simulink model "Controller"  (R2020b)
settings: Solver=VariableStepAuto  StartTime=0.0  StopTime=50  RelTol=1e-3
settings Model: Creator=Awan  LastModifiedBy=Awan
settings SolverCC: ZeroCrossAlgorithm=Adaptive
settings DebuggingCC: IgnoredZcDiagnostic=none

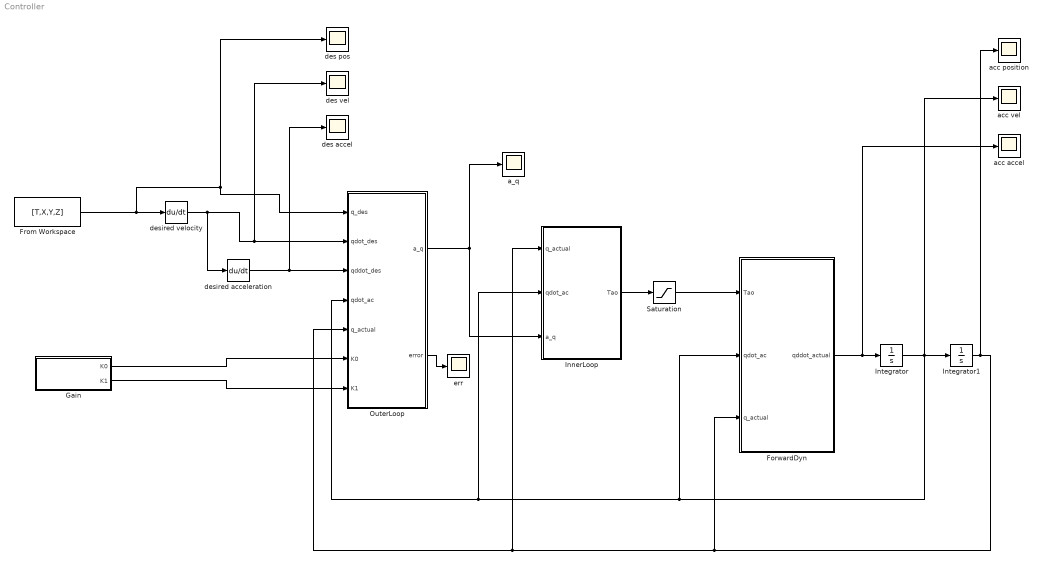
== system Controller ==
  ForwardDyn : MATLAB Function  TreatAsAtomicUnit=on
  From Workspace : FromWorkspace  VariableName=[T,X,Y,Z]
  Gain : Subsystem
  InnerLoop : MATLAB Function  TreatAsAtomicUnit=on
  Integrator : Integrator  InitialCondition=[0,0,0]
  Integrator1 : Integrator  InitialCondition=[0,0,0]
  OuterLoop : MATLAB Function  TreatAsAtomicUnit=on
  Saturation : Saturate  UpperLimit=6000  LowerLimit=-6000  ZeroCross=off
  a_q : Scope
  acc accel : Scope
  acc position : Scope
  acc vel : Scope
  des accel : Scope
  des pos : Scope
  des vel : Scope
  desired acceleration : Derivative
  desired velocity : Derivative
  err : Scope
  wires:
  desired acceleration/1 -> des accel/1, OuterLoop/3(qddot_des)
  desired velocity/1 -> desired acceleration/1, des vel/1, OuterLoop/2(qdot_des)
  Gain/1(K0) -> OuterLoop/6(K0)
  Gain/2(K1) -> OuterLoop/7(K1)
  OuterLoop/2(error) -> err/1
  From Workspace/1 -> des pos/1, OuterLoop/1(q_des), desired velocity/1
  OuterLoop/1(a_q) -> a_q/1, InnerLoop/3(a_q)
  InnerLoop/1(Tao) -> Saturation/1
  Saturation/1 -> ForwardDyn/1(Tao)
  ForwardDyn/1(qddot_actual) -> acc accel/1, Integrator/1
  Integrator/1 -> Integrator1/1, acc vel/1, InnerLoop/2(qdot_ac), OuterLoop/4(qdot_ac), ForwardDyn/2(qdot_ac)
  Integrator1/1 -> InnerLoop/1(q_actual), OuterLoop/5(q_actual), ForwardDyn/3(q_actual), acc position/1

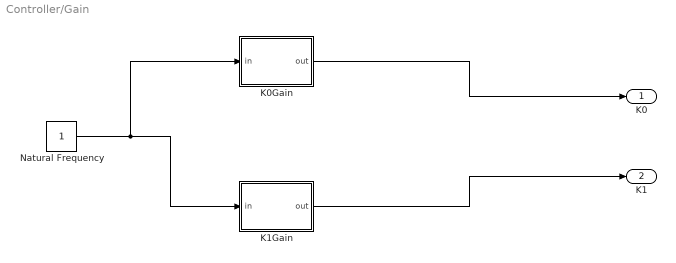
== system Controller/Gain ==
  K0Gain : MATLAB Function  TreatAsAtomicUnit=on
  K1Gain : MATLAB Function  TreatAsAtomicUnit=on
  Natural Frequency : Constant
  K0 : Outport
  K1 : Outport  Port=2  VectorParamsAs1DForOutWhenUnconnected=off
  wires:
  K1Gain/1(out) -> K1/1
  K0Gain/1(out) -> K0/1
  Natural Frequency/1 -> K1Gain/1(in), K0Gain/1(in)

== matlab function Controller/Gain/K1Gain ==
  data: in input; out output
function out = K1Gain(in)
%gain adjustment for K1
in=0.7*in;

out=[in, 0, 0; 0, in, 0; 0, 0, in];

== matlab function Controller/OuterLoop ==
  data: q_des input; a_q output; qdot_des input; qddot_des input; qdot_ac input; q_actual input; K0 input; K1 input; error output
function [a_q,error] = control(q_des,qdot_des,qddot_des,qdot_ac,q_actual,K0,K1)
%Linear System Stabilizer/Outer Loop Controller 

q_squig=(q_actual - q_des);
qdot_squig=(qdot_ac-qdot_des);

a_q = (qddot_des)-(K0*q_squig)-(K1*qdot_squig);
error = [q_des-q_actual];

== matlab function Controller/Gain/K0Gain ==
  data: in input; out output
function out = K0Gain(in)
%gain adjustment for K0
in=0.3*in;

out=[in, 0, 0; 0, in, 0; 0, 0, in];

== matlab function Controller/InnerLoop ==
  data: q_actual input; qdot_ac input; a_q input; Tao output
function Tao=dyneqoutloop(q_actual,qdot_ac,a_q) 
%Function that calculates Torques based on the Euler Lagrange Method
%Now Modified for Inner Loop
%************************************************************************
%Code Section 1: Input Parameters 
%************************************************************************
m= [945.89, 480.13, 112.70]; %mass per link (g) 
L= [1.5, 1.75, 0.3]; %link lengths (m) 
L_c=[0.65, 0.84, 0.17]; %distances from link start to centre of mass (m)
g=9.81; %grav constant 
%intertia matrices about centre of masses
I1=[ 196.52, 0, 0; 0, 53.6, 0; 0, 0, 191.83 ];
I2=[ 8.41, 0, 0; 0, 144.37, 0; 0, 0, 147.97 ];
I3=[ 3.52, 0, 0; 0, 5.10, 0; 0, 0, 3.15 ];
%************************************************************************
%Code Section 2: Computing DH Matrices 
%************************************************************************
%DH Parameters 
a = [0, L(2), L(3)]; %a values 
d = [L(1), 0, 0]; %d values 
a_c = [0, L_c(2), L_c(3)]; %a values, modified for centre of mass
d_c = [L_c(1), 0, 0]; %d values, modified for centre of mass
alpha = [-pi/2, 0, 0]; %alpha angles
theta = [q_actual(1), q_actual(2), q_actual(3)]; %joint angles
%Regulr DH Matrices  
A1= [ cos(theta(1)), -sin(theta(1)) * cosd(alpha(1)*(180/pi)), sin(theta(1))*sind(alpha(1)*(180/pi)), a(1)*cos(theta(1)); 
            sin(theta(1)), cos(theta(1))*cosd(alpha(1)*(180/pi)), -cos(theta(1))*sind(alpha(1)*(180/pi)), a(1)*sin(theta(1));
            0, sind(alpha(1)*(180/pi)), cosd(alpha(1)*(180/pi)), d(1); 
            0, 0, 0, 1; ]; 
        
Temp_A2= [ cos(theta(2)), -sin(theta(2)) * cosd(alpha(2)*(180/pi)), sin(theta(2))*sind(alpha(2)*(180/pi)), a(2)*cos(theta(2)); 
            sin(theta(2)), cos(theta(2))*cosd(alpha(2)*(180/pi)), -cos(theta(2))*sind(alpha(2)*(180/pi)), a(2)*sin(theta(2));
            0, sind(alpha(2)*(180/pi)), cosd(alpha(2)*(180/pi)), d(2); 
            0, 0, 0, 1; ]; 
        
%Modded DH Matrices  
Ac1= [ cos(theta(1)), -sin(theta(1)) * cosd(alpha(1)*(180/pi)), sin(theta(1))*sind(alpha(1)*(180/pi)), a_c(1)*cos(theta(1)); 
            sin(theta(1)), cos(theta(1))*cosd(alpha(1)*(180/pi)), -cos(theta(1))*sind(alpha(1)*(180/pi)), a_c(1)*sin(theta(1));
            0, sind(alpha(1)*(180/pi)), cosd(alpha(1)*(180/pi)), d_c(1); 
            0, 0, 0, 1; ] ;
             
Temp_Ac2= [ cos(theta(2)), -sin(theta(2)) * cosd(alpha(2)*(180/pi)), sin(theta(2))*sind(alpha(2)*(180/pi)), a_c(2)*cos(theta(2)); 
            sin(theta(2)), cos(theta(2))*cosd(alpha(2)*(180/pi)), -cos(theta(2))*sind(alpha(2)*(180/pi)), a_c(2)*sin(theta(2));
            0, sind(alpha(2)*(180/pi)), cosd(alpha(2)*(180/pi)), d_c(2); 
            0, 0, 0, 1; ] ;        
        
Temp_Ac3= [ cos(theta(3)), -sin(theta(3)) * cosd(alpha(3)*(180/pi)), sin(theta(3))*sind(alpha(3)*(180/pi)), a_c(3)*cos(theta(3)); 
            sin(theta(3)), cos(theta(3))*cosd(alpha(3)*(180/pi)), -cos(theta(3))*sind(alpha(3)*(180/pi)), a_c(3)*sin(theta(3));
            0, sind(alpha(3)*(180/pi)), cosd(alpha(3)*(180/pi)), d_c(3); 
            0, 0, 0, 1; ] ;
%Computing Transformation Matrices
A2=A1*Temp_A2;
Ac2=A1*Temp_Ac2;
Ac3=A1*Temp_A2*Temp_Ac3;
%************************************************************************
%Code Section 3: Computing Jacobian Matrices 
%************************************************************************        
%z vectors
z0=[0 0 1].';
z1= A1(1:3, 3);
z2= A2(1:3, 3);
%origin vectors
o0=[0 0 0].';
o1= A1(1:3, 4);
o2= A2(1:3, 4);
%centre of mass origin vectors 
oc1=Ac1(1:3, 4);
oc2=Ac2(1:3, 4);
oc3=Ac3(1:3, 4);
%Jacobians
J1=[ cross(z0,oc1 - o0), zeros(3,1), zeros(3,1);
     z0, zeros(3,1), zeros(3,1) ];
J2=[ cross(z0,oc2 - o0), cross(z1,oc2 - o1), zeros(3,1);
    z0, z1, zeros(3,1) ];
J3=[ cross(z0,oc3 - o0), cross(z1,oc3 - o1), cross(z2,oc3 - o2);
    z0, z1, z2 ];        
%************************************************************************
%Code Section 4: Computing Linear and Rotational Kinetic Energy
%************************************************************************
%Velocity Jacobians 
Jv1=J1(1:3,1:3);
Jv2=J2(1:3,1:3);
Jv3=J3(1:3,1:3);
%Linear KE Calculation
KL1=m(1)*(Jv1.')*Jv1;
KL2=m(2)*(Jv2.')*Jv2;
KL3=m(3)*(Jv3.')*Jv3;
%************************************************************************
%Rotational Jacobians 
Jw1=J1(4:6,1:3);
Jw2=J2(4:6,1:3);
Jw3=J3(4:6,1:3);
%R values 
R1=Ac1(1:3,1:3);
R2=Ac2(1:3,1:3);
R3=Ac3(1:3,1:3);
%Rotational KE Calculation
KW1=(Jw1.')*R1*I1*(R1.')*Jw1;
KW2=(Jw2.')*R2*I2*(R2.')*Jw2;
KW3=(Jw3.')*R3*I3*(R3.')*Jw3;
%************************************************************************
%Code Section 5: Computing Inertia Matrix
%************************************************************************
%Summing Kinetic Energies
SumKE1=KL1*KW1;
SumKE2=KL2*KW2;
SumKE3=KL3*KW3;
%Formulating D Matrix 
D=SumKE1+SumKE2+SumKE3;
%************************************************************************
%Code Section 6: Computing Christoffel Symbols (Modified and Taken from EulerLagrangeAttempt2.m 
%************************************************************************
%cij1 values 
c111=0;
c221=0;
c331=0;

c121=- 157.7504*sin(2*q_actual(2) + q_actual(3)) - 2.5199e+04*sin(2*q_actual(2)) - 1.1515e+04*sin(4*q_actual(2)) - 144.6372*sin(2*q_actual(2) + 2*q_actual(3)) - 13.2437*sin(2*q_actual(2) + 3*q_actual(3)) - 136.3318*sin(4*q_actual(2) + 2*q_actual(3)) - 26.4873*sin(4*q_actual(2) + 3*q_actual(3)) - 1.2865*sin(4*q_actual(2) + 4*q_actual(3));
c131=- 78.8752*sin(2*q_actual(2) + q_actual(3)) - 68.1659*sin(2*q_actual(3)) - 144.6372*sin(2*q_actual(2) + 2*q_actual(3)) - 19.8655*sin(2*q_actual(2) + 3*q_actual(3)) - 68.1659*sin(4*q_actual(2) + 2*q_actual(3)) - 19.8655*sin(4*q_actual(2) + 3*q_actual(3)) - 1.2865*sin(4*q_actual(2) + 4*q_actual(3)) - 78.8752*sin(q_actual(3));

c211=c121;
c311=c131;

c231=0;
c321=c231;

%cij2 values 
c112=157.7504*sin(2*q_actual(2) + q_actual(3)) + 2.5199e+04*sin(2*q_actual(2)) + 1.1515e+04*sin(4*q_actual(2)) + 144.6372*sin(2*q_actual(2) + 2*q_actual(3)) + 13.2437*sin(2*q_actual(2) + 3*q_actual(3)) + 136.3318*sin(4*q_actual(2) + 2*q_actual(3)) + 26.4873*sin(4*q_actual(2) + 3*q_actual(3)) + 1.2865*sin(4*q_actual(2) + 4*q_actual(3));
c222=0;
c332=-316.8420*sin(q_actual(3));

c122=157.7504*sin(2*q_actual(2) + q_actual(3)) + 2.5199e+04*sin(2*q_actual(2)) + 1.1515e+04*sin(4*q_actual(2)) + 144.6372*sin(2*q_actual(2) + 2*q_actual(3)) + 13.2437*sin(2*q_actual(2) + 3*q_actual(3)) + 136.3318*sin(4*q_actual(2) + 2*q_actual(3)) + 26.4873*sin(4*q_actual(2) + 3*q_actual(3)) + 1.2865*sin(4*q_actual(2) + 4*q_actual(3));
c132=157.7504*sin(2*q_actual(2) + q_actual(3)) + 2.5199e+04*sin(2*q_actual(2)) + 1.1515e+04*sin(4*q_actual(2)) + 144.6372*sin(2*q_actual(2) + 2*q_actual(3)) + 13.2437*sin(2*q_actual(2) + 3*q_actual(3)) + 136.3318*sin(4*q_actual(2) + 2*q_actual(3)) + 26.4873*sin(4*q_actual(2) + 3*q_actual(3)) + 1.2865*sin(4*q_actual(2) + 4*q_actual(3));

c212=c122;
c312=c132;

c232=-158.4210*sin(q_actual(3));
c322=c232;

%cij3 values 
c113=78.8752*sin(2*q_actual(2) + q_actual(3)) + 68.1659*sin(2*q_actual(3)) + 144.6372*sin(2*q_actual(2) + 2*q_actual(3)) + 19.8655*sin(2*q_actual(2) + 3*q_actual(3)) + 68.1659*sin(4*q_actual(2) + 2*q_actual(3)) + 19.8655*sin(4*q_actual(2) + 3*q_actual(3)) + 1.2865*sin(4*q_actual(2) + 4*q_actual(3)) + 78.8752*sin(q_actual(3));
c223=158.4210*sin(q_actual(3));
c333=-52.8070*sin(q_actual(3));

c123=78.8752*sin(2*q_actual(2) + q_actual(3)) + 68.1659*sin(2*q_actual(3)) + 144.6372*sin(2*q_actual(2) + 2*q_actual(3)) + 19.8655*sin(2*q_actual(2) + 3*q_actual(3)) + 68.1659*sin(4*q_actual(2) + 2*q_actual(3)) + 19.8655*sin(4*q_actual(2) + 3*q_actual(3)) + 1.2865*sin(4*q_actual(2) + 4*q_actual(3)) + 78.8752*sin(q_actual(3));
c133=78.8752*sin(2*q_actual(2) + q_actual(3)) + 68.1659*sin(2*q_actual(3)) + 144.6372*sin(2*q_actual(2) + 2*q_actual(3)) + 19.8655*sin(2*q_actual(2) + 3*q_actual(3)) + 68.1659*sin(4*q_actual(2) + 2*q_actual(3)) + 19.8655*sin(4*q_actual(2) + 3*q_actual(3)) + 1.2865*sin(4*q_actual(2) + 4*q_actual(3)) + 78.8752*sin(q_actual(3));


c213=c123;
c313=c133;

c233=0;
c323=c233;
%************************************************************************
%C matrices
C1_temp=[c111, c211, c311; c121, c221, c321; c131, c231, c331];
C2_temp=[c112, c212, c312; c122, c222, c322; c132, c232, c332];
C3_temp=[c113, c213, c313; c123, c223, c323; c133, c233, c333];

C1=C1_temp;
C2=C2_temp;
C3=C3_temp;
%************************************************************************
%Code Section 7: Computing Potential Energy Gradient  
%************************************************************************
%Potential Energy Calculation
%g values
g1=0;
g2=-3.9565e+03*cos(q_actual(2));
g3=187.9498*sin(q_actual(2))*sin(q_actual(3)) - 187.9498*cos(q_actual(2))*cos(q_actual(3));
%Formulating G matrix
G=[g1 g2 g3].';
%************************************************************************
%Code Section 8: Bringing it all together and Computing Tao  
%************************************************************************        
%Computing Individual Tao Terms 
Term1=(D*a_q);
Term2=((([C1*qdot_ac,C2*qdot_ac,C3*qdot_ac].')*qdot_ac));
Term3=G;
%Summation and Simplification of Tao Terms 
Tao=Term1+Term2+Term3; 
%************************************************************************
%End of function  
%************************************************************************

== matlab function Controller/ForwardDyn ==
  data: Tao input; qddot_actual output; qdot_ac input; q_actual input
function qddot_actual= dyneqfordyn(Tao,qdot_ac,q_actual)
%Function that calculates Torques based on the Euler Lagrange Method
%Modified for Forward Dyn Controller
%************************************************************************
%Code Section 1: Input Parameters 
%************************************************************************
m= [945.89, 480.13, 112.70]; %mass per link (g) 
L= [1.5, 1.75, 0.3]; %link lengths (m) 
L_c=[0.65, 0.84, 0.17]; %distances from link start to centre of mass (m)
g=9.81; %grav constant 
%intertia matrices about centre of masses
I1=[ 196.52, 0, 0; 0, 53.6, 0; 0, 0, 191.83 ];
I2=[ 8.41, 0, 0; 0, 144.37, 0; 0, 0, 147.97 ];
I3=[ 3.52, 0, 0; 0, 5.10, 0; 0, 0, 3.15 ];
%************************************************************************
%Code Section 2: Computing DH Matrices 
%************************************************************************
%DH Parameters 
a = [0, L(2), L(3)]; %a values 
d = [L(1), 0, 0]; %d values 
a_c = [0, L_c(2), L_c(3)]; %a values, modified for centre of mass
d_c = [L_c(1), 0, 0]; %d values, modified for centre of mass
alpha = [-pi/2, 0, 0]; %alpha angles
theta = [q_actual(1), q_actual(2), q_actual(3)]; %joint angles
%Regulr DH Matrices  
A1= [ cos(theta(1)), -sin(theta(1)) * cosd(alpha(1)*(180/pi)), sin(theta(1))*sind(alpha(1)*(180/pi)), a(1)*cos(theta(1)); 
            sin(theta(1)), cos(theta(1))*cosd(alpha(1)*(180/pi)), -cos(theta(1))*sind(alpha(1)*(180/pi)), a(1)*sin(theta(1));
            0, sind(alpha(1)*(180/pi)), cosd(alpha(1)*(180/pi)), d(1); 
            0, 0, 0, 1; ]; 
        
Temp_A2= [ cos(theta(2)), -sin(theta(2)) * cosd(alpha(2)*(180/pi)), sin(theta(2))*sind(alpha(2)*(180/pi)), a(2)*cos(theta(2)); 
            sin(theta(2)), cos(theta(2))*cosd(alpha(2)*(180/pi)), -cos(theta(2))*sind(alpha(2)*(180/pi)), a(2)*sin(theta(2));
            0, sind(alpha(2)*(180/pi)), cosd(alpha(2)*(180/pi)), d(2); 
            0, 0, 0, 1; ]; 
        
%Modded DH Matrices  
Ac1= [ cos(theta(1)), -sin(theta(1)) * cosd(alpha(1)*(180/pi)), sin(theta(1))*sind(alpha(1)*(180/pi)), a_c(1)*cos(theta(1)); 
            sin(theta(1)), cos(theta(1))*cosd(alpha(1)*(180/pi)), -cos(theta(1))*sind(alpha(1)*(180/pi)), a_c(1)*sin(theta(1));
            0, sind(alpha(1)*(180/pi)), cosd(alpha(1)*(180/pi)), d_c(1); 
            0, 0, 0, 1; ] ;
             
Temp_Ac2= [ cos(theta(2)), -sin(theta(2)) * cosd(alpha(2)*(180/pi)), sin(theta(2))*sind(alpha(2)*(180/pi)), a_c(2)*cos(theta(2)); 
            sin(theta(2)), cos(theta(2))*cosd(alpha(2)*(180/pi)), -cos(theta(2))*sind(alpha(2)*(180/pi)), a_c(2)*sin(theta(2));
            0, sind(alpha(2)*(180/pi)), cosd(alpha(2)*(180/pi)), d_c(2); 
            0, 0, 0, 1; ] ;        
        
Temp_Ac3= [ cos(theta(3)), -sin(theta(3)) * cosd(alpha(3)*(180/pi)), sin(theta(3))*sind(alpha(3)*(180/pi)), a_c(3)*cos(theta(3)); 
            sin(theta(3)), cos(theta(3))*cosd(alpha(3)*(180/pi)), -cos(theta(3))*sind(alpha(3)*(180/pi)), a_c(3)*sin(theta(3));
            0, sind(alpha(3)*(180/pi)), cosd(alpha(3)*(180/pi)), d_c(3); 
            0, 0, 0, 1; ] ;
%Computing Transformation Matrices
A2=A1*Temp_A2;
Ac2=A1*Temp_Ac2;
Ac3=A1*Temp_A2*Temp_Ac3;
%************************************************************************
%Code Section 3: Computing Jacobian Matrices 
%************************************************************************        
%z vectors
z0=[0 0 1].';
z1= A1(1:3, 3);
z2= A2(1:3, 3);
%origin vectors
o0=[0 0 0].';
o1= A1(1:3, 4);
o2= A2(1:3, 4);
%centre of mass origin vectors 
oc1=Ac1(1:3, 4);
oc2=Ac2(1:3, 4);
oc3=Ac3(1:3, 4);
%Jacobians
J1=[ cross(z0,oc1 - o0), zeros(3,1), zeros(3,1);
     z0, zeros(3,1), zeros(3,1) ];
J2=[ cross(z0,oc2 - o0), cross(z1,oc2 - o1), zeros(3,1);
    z0, z1, zeros(3,1) ];
J3=[ cross(z0,oc3 - o0), cross(z1,oc3 - o1), cross(z2,oc3 - o2);
    z0, z1, z2 ];        
%************************************************************************
%Code Section 4: Computing Linear and Rotational Kinetic Energy
%************************************************************************
%Velocity Jacobians 
Jv1=J1(1:3,1:3);
Jv2=J2(1:3,1:3);
Jv3=J3(1:3,1:3);
%Linear KE Calculation
KL1=m(1)*(Jv1.')*Jv1;
KL2=m(2)*(Jv2.')*Jv2;
KL3=m(3)*(Jv3.')*Jv3;
%************************************************************************
%Rotational Jacobians 
Jw1=J1(4:6,1:3);
Jw2=J2(4:6,1:3);
Jw3=J3(4:6,1:3);
%R values 
R1=Ac1(1:3,1:3);
R2=Ac2(1:3,1:3);
R3=Ac3(1:3,1:3);
%Rotational KE Calculation
KW1=(Jw1.')*R1*I1*(R1.')*Jw1;
KW2=(Jw2.')*R2*I2*(R2.')*Jw2;
KW3=(Jw3.')*R3*I3*(R3.')*Jw3;
%************************************************************************
%Code Section 5: Computing Inertia Matrix
%************************************************************************
%Summing Kinetic Energies
SumKE1=KL1*KW1;
SumKE2=KL2*KW2;
SumKE3=KL3*KW3;
%Formulating D Matrix 
D=SumKE1+SumKE2+SumKE3;
%************************************************************************
%Code Section 6: Computing Christoffel Symbols (Modified and Taken from EulerLagrangeAttempt2.m 
%************************************************************************
%cij1 values 
c111=0;
c221=0;
c331=0;

c121=- 157.7504*sin(2*q_actual(2) + q_actual(3)) - 2.5199e+04*sin(2*q_actual(2)) - 1.1515e+04*sin(4*q_actual(2)) - 144.6372*sin(2*q_actual(2) + 2*q_actual(3)) - 13.2437*sin(2*q_actual(2) + 3*q_actual(3)) - 136.3318*sin(4*q_actual(2) + 2*q_actual(3)) - 26.4873*sin(4*q_actual(2) + 3*q_actual(3)) - 1.2865*sin(4*q_actual(2) + 4*q_actual(3));
c131=- 78.8752*sin(2*q_actual(2) + q_actual(3)) - 68.1659*sin(2*q_actual(3)) - 144.6372*sin(2*q_actual(2) + 2*q_actual(3)) - 19.8655*sin(2*q_actual(2) + 3*q_actual(3)) - 68.1659*sin(4*q_actual(2) + 2*q_actual(3)) - 19.8655*sin(4*q_actual(2) + 3*q_actual(3)) - 1.2865*sin(4*q_actual(2) + 4*q_actual(3)) - 78.8752*sin(q_actual(3));

c211=c121;
c311=c131;

c231=0;
c321=c231;

%cij2 values 
c112=157.7504*sin(2*q_actual(2) + q_actual(3)) + 2.5199e+04*sin(2*q_actual(2)) + 1.1515e+04*sin(4*q_actual(2)) + 144.6372*sin(2*q_actual(2) + 2*q_actual(3)) + 13.2437*sin(2*q_actual(2) + 3*q_actual(3)) + 136.3318*sin(4*q_actual(2) + 2*q_actual(3)) + 26.4873*sin(4*q_actual(2) + 3*q_actual(3)) + 1.2865*sin(4*q_actual(2) + 4*q_actual(3));
c222=0;
c332=-316.8420*sin(q_actual(3));

c122=157.7504*sin(2*q_actual(2) + q_actual(3)) + 2.5199e+04*sin(2*q_actual(2)) + 1.1515e+04*sin(4*q_actual(2)) + 144.6372*sin(2*q_actual(2) + 2*q_actual(3)) + 13.2437*sin(2*q_actual(2) + 3*q_actual(3)) + 136.3318*sin(4*q_actual(2) + 2*q_actual(3)) + 26.4873*sin(4*q_actual(2) + 3*q_actual(3)) + 1.2865*sin(4*q_actual(2) + 4*q_actual(3));
c132=157.7504*sin(2*q_actual(2) + q_actual(3)) + 2.5199e+04*sin(2*q_actual(2)) + 1.1515e+04*sin(4*q_actual(2)) + 144.6372*sin(2*q_actual(2) + 2*q_actual(3)) + 13.2437*sin(2*q_actual(2) + 3*q_actual(3)) + 136.3318*sin(4*q_actual(2) + 2*q_actual(3)) + 26.4873*sin(4*q_actual(2) + 3*q_actual(3)) + 1.2865*sin(4*q_actual(2) + 4*q_actual(3));

c212=c122;
c312=c132;

c232=-158.4210*sin(q_actual(3));
c322=c232;

%cij3 values 
c113=78.8752*sin(2*q_actual(2) + q_actual(3)) + 68.1659*sin(2*q_actual(3)) + 144.6372*sin(2*q_actual(2) + 2*q_actual(3)) + 19.8655*sin(2*q_actual(2) + 3*q_actual(3)) + 68.1659*sin(4*q_actual(2) + 2*q_actual(3)) + 19.8655*sin(4*q_actual(2) + 3*q_actual(3)) + 1.2865*sin(4*q_actual(2) + 4*q_actual(3)) + 78.8752*sin(q_actual(3));
c223=158.4210*sin(q_actual(3));
c333=-52.8070*sin(q_actual(3));

c123=78.8752*sin(2*q_actual(2) + q_actual(3)) + 68.1659*sin(2*q_actual(3)) + 144.6372*sin(2*q_actual(2) + 2*q_actual(3)) + 19.8655*sin(2*q_actual(2) + 3*q_actual(3)) + 68.1659*sin(4*q_actual(2) + 2*q_actual(3)) + 19.8655*sin(4*q_actual(2) + 3*q_actual(3)) + 1.2865*sin(4*q_actual(2) + 4*q_actual(3)) + 78.8752*sin(q_actual(3));
c133=78.8752*sin(2*q_actual(2) + q_actual(3)) + 68.1659*sin(2*q_actual(3)) + 144.6372*sin(2*q_actual(2) + 2*q_actual(3)) + 19.8655*sin(2*q_actual(2) + 3*q_actual(3)) + 68.1659*sin(4*q_actual(2) + 2*q_actual(3)) + 19.8655*sin(4*q_actual(2) + 3*q_actual(3)) + 1.2865*sin(4*q_actual(2) + 4*q_actual(3)) + 78.8752*sin(q_actual(3));


c213=c123;
c313=c133;

c233=0;
c323=c233;
%************************************************************************
%C matrices
C1_temp=[c111, c211, c311; c121, c221, c321; c131, c231, c331];
C2_temp=[c112, c212, c312; c122, c222, c322; c132, c232, c332];
C3_temp=[c113, c213, c313; c123, c223, c323; c133, c233, c333];

C1=C1_temp;
C2=C2_temp;
C3=C3_temp;
%************************************************************************
%Code Section 7: Computing Potential Energy Gradient  
%************************************************************************
%Potential Energy Calculation
%g values
g1=0;
g2=-3.9565e+03*cos(q_actual(2));
g3=187.9498*sin(q_actual(2))*sin(q_actual(3)) - 187.9498*cos(q_actual(2))*cos(q_actual(3));
%Formulating G matrix
G=[g1 g2 g3].';
%************************************************************************
%Code Section 8: Bringing it all together and Computing Tao  
%************************************************************************        
%Computing Individual Tao Terms 
Term1=inv(D);
Term2=((([C1*qdot_ac,C2*qdot_ac,C3*qdot_ac].')*qdot_ac));
Term3=G;

qddot_actual=Term1*(Tao-Term2-Term3);
%************************************************************************
%End of function  
%************************************************************************
